simulink model "closed_loop"  (R2025b)
settings: Solver=VariableStepAuto  StartTime=0.0  StopTime=10.0  RelTol=1e-3
values from neighbouring files (symbols this model uses):
  A = [0, 0, 1, 0 ... (first row only)    [inv_pend.m]
  B = [0; 0; (Km*Kg)/(M*Rm*r); (-Km*Kg)/(r*Rm*M*l)]    [inv_pend.m]
  K = lqr(A, B, Q, R)    [inv_pend.m]
settings Model: Creator=sm  LastModifiedBy=sm

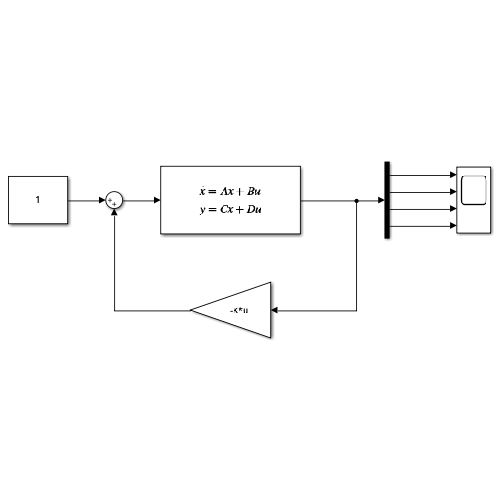
[thumbnail: Simulink's stored preview of the top-level diagram]
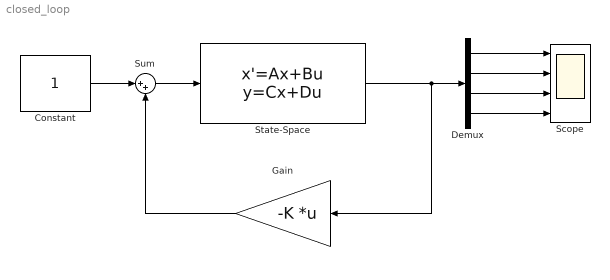
== system closed_loop ==
  Constant : Constant
  Demux : Demux
  Gain : Gain  Gain=-K  Multiplication=Matrix(K*u)
  Scope : Scope  NumInputPorts=4
      settings: ActiveDisplayString=4  Title=Angular Velocity [rad/s]  ActiveDisplayYMinimum=-0.24107674099007842  ActiveDisplayYMaximum=0.0797599942448491
  State-Space : StateSpace  A=A  B=B  C=eye(4)  D=zeros(4,1)  InitialCondition=[0; 0; 0; 0]
  Sum : Sum  Inputs=|++
  wires:
  Demux/4 -> Scope/4
  Demux/2 -> Scope/2
  Demux/1 -> Scope/1
  Constant/1 -> Sum/1
  Demux/3 -> Scope/3
  State-Space/1 -> Gain/1, Demux/1
  Gain/1 -> Sum/2
  Sum/1 -> State-Space/1
